simulink model "Microgrid_W"  (R2020a)
settings: Solver=ode15s  StartTime=0  StopTime=1440*1  MaxStep=1  RelTol=1e-3
libraries: simulink x4214, powerlib x685, simulink_extras x28, Microgrid_Library x18, powerlib_meascontrol x12
(part 2 of 48)

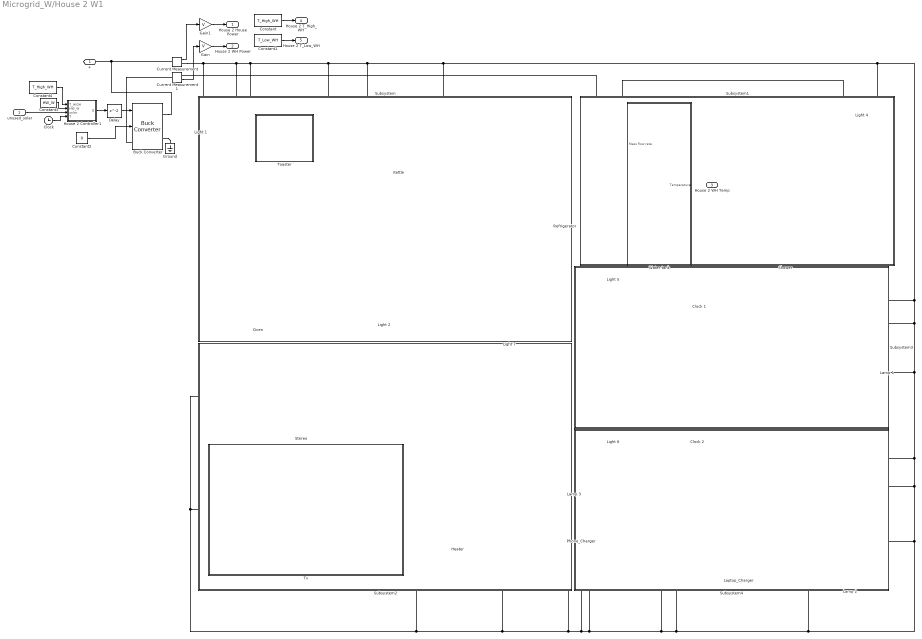
== system Microgrid_W/House 2 W1 ==
  unused_solar : Inport
  Buck Converter : powerlib/Power Electronics/Buck Converter  ModelType=Average model (D-controlled)  Ron=1e-3  Rs=1e6  Cs=inf  Vforward=[0,0]  Ron_Diode=1e-3  Rs_Diode=1e6  Cs_Diode=inf  Vf_Diode=1e-3  Rs_CurrentSource=inf
      settings: SourceProductBaseCode=PS
  Clock : Clock
  Clock 1 : Subsystem
      mask Display: image('Clock.jpg');
  Clock 2 : Subsystem
      mask Display: image('Clock.jpg');
  Constant : Constant  Value=T_High_WH
  Constant1 : Constant  Value=T_Low_WH
  Constant2 : Constant  Value=0
  Constant3 : Constant  Value=HW_W
  Constant4 : Constant  Value=T_High_WH
  Current Measurement : powerlib/Measurements/Current Measurement  PhasorSimulation=off  OutputType=Complex  PSBequivalent=0
  Current Measurement1 : powerlib/Measurements/Current Measurement  PhasorSimulation=off  OutputType=Complex  PSBequivalent=0
  Delay : Delay
  Gain : Gain  Gain=V
  Gain1 : Gain  Gain=V
  Ground : powerlib/Elements/Ground  LConnTagsString=a
  Heater : Subsystem
      mask Display: image('oil_heater.jpg');
  House 2 Controller1 : MATLAB Function  TreatAsAtomicUnit=on
  Kettle : Subsystem
      mask Display: image('jug.jpg');
  Lamp 1 : Subsystem
      mask Display: image('Lamp_1.jpg');
  Lamp 2 : Subsystem
      mask Display: image('Lamp_1.jpg');
  Lamp 3 : Subsystem
      mask Display: image('Lamp_1.jpg');
  Laptop_Charger : Subsystem
      mask Display: image('Laptop.jpg');
  Light 1 : Subsystem
      mask Display: image('LightBulb.jpg');
  Light 2 : Subsystem
      mask Display: image('Dishwasher.jpg');
  Light 4 : Subsystem
      mask Display: image('LightBulb.jpg');
  Light 5 : Subsystem
      mask Display: image('LightBulb.jpg');
  Light 6 : Subsystem
      mask Display: image('LightBulb.jpg');
  Light 7 : Subsystem
      mask Display: image('LightBulb.jpg');
  Oven : Subsystem
      mask Display: image('oven.jpg');
  Phone_Charger : Subsystem
      mask Display: image('Phone.jpg');
  Refrigerator : Subsystem
      mask Display: image('firdge1.JPG');
  Shower : Subsystem
      mask Display: image('Shower.jpg');
  Stereo : Subsystem
      mask Display: image('Stereo.jpg');
  Subsystem : Subsystem
      mask Display: patch([1 1 0 0],[1 0 0 1], [1, .4, .4])
  Subsystem1 : Subsystem
      mask Display: patch([1 1 0 0],[1 0 0 1], [0.6, .8, 1])
  Subsystem2 : Subsystem
      mask Display: patch([1 1 0 0],[1 0 0 1], [0.4, 1, .4])
  Subsystem3 : Subsystem
      mask Display: patch([1 1 0 0],[1 0 0 1], [0.8, 0.42, 0])
  Subsystem4 : Subsystem
      mask Display: patch([1 1 0 0],[1 0 0 1], [0.75, .75, .75])
  Toaster : Subsystem
      mask Display: image('toaster.jpg');
  Tv : Subsystem
      mask Display: image('Tel.jpg');
  Water tank : Subsystem
      mask Display: image('Hot Water.jpg');
  + : PMIOPort  Side=Left
  House 2 House Power : Outport
  House 2 WH Power : Outport  Port=2
  House 2 WH Temp : Outport  Port=3
  House 2 T_High_WH : Outport  Port=4
  House 2 T_Low_WH : Outport  Port=5
  wires:
  Shower/1(Out1) -> Water tank/1(Mass flow rate)
  Water tank/1(Temperature) -> House 2 WH Temp/1
  Constant/1 -> House 2 T_High_WH/1
  Constant1/1 -> House 2 T_Low_WH/1
  Current Measurement1/1 -> Gain/1
  Current Measurement/1 -> Gain1/1
  Gain1/1 -> House 2 House Power/1
  Constant2/1 -> Buck Converter/2
  Constant3/1 -> House 2 Controller1/2(HW_W)
  House 2 Controller1/1(D) -> Delay/1
  Delay/1 -> Buck Converter/1
  Clock/1 -> House 2 Controller1/4(T)
  unused_solar/1 -> House 2 Controller1/3(solar)
  Gain/1 -> House 2 WH Power/1
  Constant4/1 -> House 2 Controller1/1(T_HIGH)
  connections:
  Buck Converter/LConn1 -- Current Measurement1/LConn1
  Light 1/LConn1 -- Oven/LConn1 -- Current Measurement/RConn1 -- Light 4/LConn1 -- Light 5/LConn1 -- Clock 1/LConn1 -- Lamp 1/LConn1 -- Clock 2/LConn1 -- Light 6/LConn1 -- Lamp 2/LConn1 -- Laptop_Charger/RConn1 -- Laptop_Charger/LConn1 -- Phone_Charger/RConn1 -- Phone_Charger/LConn2 -- Phone_Charger/LConn1 -- Light 7/LConn1 -- Lamp 3/LConn1 -- Stereo/LConn1 -- Tv/LConn1 -- Heater/LConn1 -- Refrigerator/LConn1 -- Kettle/LConn1 -- Light 2/LConn1 -- Toaster/LConn1
  Water tank/LConn1 -- Current Measurement1/RConn1
  Current Measurement/LConn1 -- Buck Converter/RConn1 -- +/RConn1
  Buck Converter/RConn2 -- Ground/LConn1

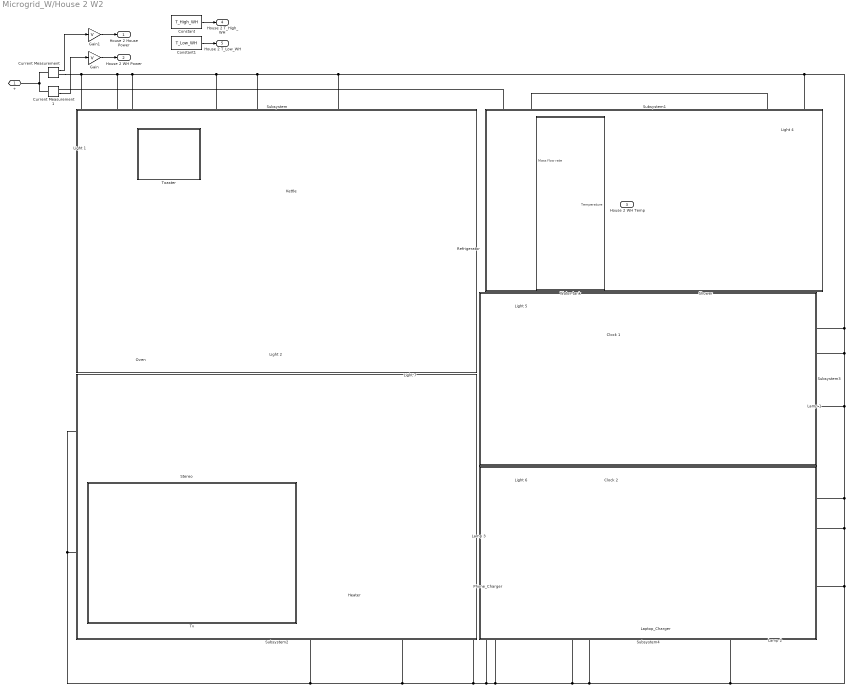
== system Microgrid_W/House 2 W2 ==
  Clock 1 : Subsystem
      mask Display: image('Clock.jpg');
  Clock 2 : Subsystem
      mask Display: image('Clock.jpg');
  Constant : Constant  Value=T_High_WH
  Constant1 : Constant  Value=T_Low_WH
  Current Measurement : powerlib/Measurements/Current Measurement  PhasorSimulation=off  OutputType=Complex  PSBequivalent=0
  Current Measurement1 : powerlib/Measurements/Current Measurement  PhasorSimulation=off  OutputType=Complex  PSBequivalent=0
  Gain : Gain  Gain=V
  Gain1 : Gain  Gain=V
  Heater : Subsystem
      mask Display: image('oil_heater.jpg');
  Kettle : Subsystem
      mask Display: image('jug.jpg');
  Lamp 1 : Subsystem
      mask Display: image('Lamp_1.jpg');
  Lamp 2 : Subsystem
      mask Display: image('Lamp_1.jpg');
  Lamp 3 : Subsystem
      mask Display: image('Lamp_1.jpg');
  Laptop_Charger : Subsystem
      mask Display: image('Laptop.jpg');
  Light 1 : Subsystem
      mask Display: image('LightBulb.jpg');
  Light 2 : Subsystem
      mask Display: image('Dishwasher.jpg');
  Light 4 : Subsystem
      mask Display: image('LightBulb.jpg');
  Light 5 : Subsystem
      mask Display: image('LightBulb.jpg');
  Light 6 : Subsystem
      mask Display: image('LightBulb.jpg');
  Light 7 : Subsystem
      mask Display: image('LightBulb.jpg');
  Oven : Subsystem
      mask Display: image('oven.jpg');
  Phone_Charger : Subsystem
      mask Display: image('Phone.jpg');
  Refrigerator : Subsystem
      mask Display: image('firdge1.JPG');
  Shower : Subsystem
      mask Display: image('Shower.jpg');
  Stereo : Subsystem
      mask Display: image('Stereo.jpg');
  Subsystem : Subsystem
      mask Display: patch([1 1 0 0],[1 0 0 1], [1, .4, .4])
  Subsystem1 : Subsystem
      mask Display: patch([1 1 0 0],[1 0 0 1], [0.6, .8, 1])
  Subsystem2 : Subsystem
      mask Display: patch([1 1 0 0],[1 0 0 1], [0.4, 1, .4])
  Subsystem3 : Subsystem
      mask Display: patch([1 1 0 0],[1 0 0 1], [0.8, 0.42, 0])
  Subsystem4 : Subsystem
      mask Display: patch([1 1 0 0],[1 0 0 1], [0.75, .75, .75])
  Toaster : Subsystem
      mask Display: image('toaster.jpg');
  Tv : Subsystem
      mask Display: image('Tel.jpg');
  Water tank : Subsystem
      mask Display: image('Hot Water.jpg');
  + : PMIOPort  Side=Left
  House 2 House Power : Outport
  House 2 WH Power : Outport  Port=2
  House 2 WH Temp : Outport  Port=3
  House 2 T_High_WH : Outport  Port=4
  House 2 T_Low_WH : Outport  Port=5
  wires:
  Shower/1(Out1) -> Water tank/1(Mass flow rate)
  Water tank/1(Temperature) -> House 2 WH Temp/1
  Constant/1 -> House 2 T_High_WH/1
  Constant1/1 -> House 2 T_Low_WH/1
  Current Measurement1/1 -> Gain/1
  Gain/1 -> House 2 WH Power/1
  Current Measurement/1 -> Gain1/1
  Gain1/1 -> House 2 House Power/1
  connections:
  Light 1/LConn1 -- Oven/LConn1 -- Current Measurement/RConn1 -- Light 4/LConn1 -- Light 5/LConn1 -- Clock 1/LConn1 -- Lamp 1/LConn1 -- Clock 2/LConn1 -- Light 6/LConn1 -- Lamp 2/LConn1 -- Laptop_Charger/RConn1 -- Laptop_Charger/LConn1 -- Phone_Charger/RConn1 -- Phone_Charger/LConn2 -- Phone_Charger/LConn1 -- Light 7/LConn1 -- Lamp 3/LConn1 -- Stereo/LConn1 -- Tv/LConn1 -- Heater/LConn1 -- Refrigerator/LConn1 -- Kettle/LConn1 -- Light 2/LConn1 -- Toaster/LConn1
  Water tank/LConn1 -- Current Measurement1/RConn1
  Current Measurement1/LConn1 -- Current Measurement/LConn1 -- +/RConn1

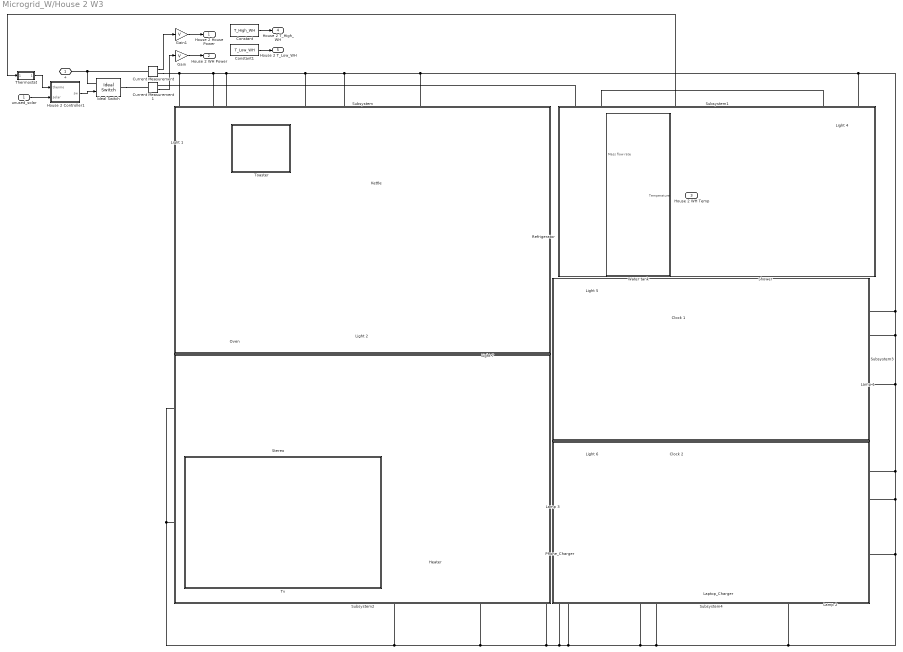
== system Microgrid_W/House 2 W3 ==
  unused_solar : Inport
  Clock 1 : Subsystem
      mask Display: image('Clock.jpg');
  Clock 2 : Subsystem
      mask Display: image('Clock.jpg');
  Constant : Constant  Value=T_High_WH
  Constant1 : Constant  Value=T_Low_WH
  Current Measurement : powerlib/Measurements/Current Measurement  PhasorSimulation=off  OutputType=Complex  PSBequivalent=0
  Current Measurement1 : powerlib/Measurements/Current Measurement  PhasorSimulation=off  OutputType=Complex  PSBequivalent=0
  Gain : Gain  Gain=V
  Gain1 : Gain  Gain=V
  Heater : Subsystem
      mask Display: image('oil_heater.jpg');
  House 2 Controller1 : MATLAB Function  TreatAsAtomicUnit=on
  Ideal Switch : powerlib/Power Electronics/Ideal Switch  Ron=0  Lon=0  IC=0  Rs=1e5  Cs=inf  Measurements=off
  Kettle : Subsystem
      mask Display: image('jug.jpg');
  Lamp 1 : Subsystem
      mask Display: image('Lamp_1.jpg');
  Lamp 2 : Subsystem
      mask Display: image('Lamp_1.jpg');
  Lamp 3 : Subsystem
      mask Display: image('Lamp_1.jpg');
  Laptop_Charger : Subsystem
      mask Display: image('Laptop.jpg');
  Light 1 : Subsystem
      mask Display: image('LightBulb.jpg');
  Light 2 : Subsystem
      mask Display: image('Dishwasher.jpg');
  Light 4 : Subsystem
      mask Display: image('LightBulb.jpg');
  Light 5 : Subsystem
      mask Display: image('LightBulb.jpg');
  Light 6 : Subsystem
      mask Display: image('LightBulb.jpg');
  Light 7 : Subsystem
      mask Display: image('LightBulb.jpg');
  Oven : Subsystem
      mask Display: image('oven.jpg');
  Phone_Charger : Subsystem
      mask Display: image('Phone.jpg');
  Refrigerator : Subsystem
      mask Display: image('firdge1.JPG');
  Shower : Subsystem
      mask Display: image('Shower.jpg');
  Stereo : Subsystem
      mask Display: image('Stereo.jpg');
  Subsystem : Subsystem
      mask Display: patch([1 1 0 0],[1 0 0 1], [1, .4, .4])
  Subsystem1 : Subsystem
      mask Display: patch([1 1 0 0],[1 0 0 1], [0.6, .8, 1])
  Subsystem2 : Subsystem
      mask Display: patch([1 1 0 0],[1 0 0 1], [0.4, 1, .4])
  Subsystem3 : Subsystem
      mask Display: patch([1 1 0 0],[1 0 0 1], [0.8, 0.42, 0])
  Subsystem4 : Subsystem
      mask Display: patch([1 1 0 0],[1 0 0 1], [0.75, .75, .75])
  Thermostat : Subsystem
  Toaster : Subsystem
      mask Display: image('toaster.jpg');
  Tv : Subsystem
      mask Display: image('Tel.jpg');
  Water tank : Subsystem
      mask Display: image('Hot Water.jpg');
  + : PMIOPort  Side=Left
  House 2 House Power : Outport
  House 2 WH Power : Outport  Port=2
  House 2 WH Temp : Outport  Port=3
  House 2 T_High_WH : Outport  Port=4
  House 2 T_Low_WH : Outport  Port=5
  wires:
  Gain1/1 -> House 2 House Power/1
  Current Measurement/1 -> Gain1/1
  Gain/1 -> House 2 WH Power/1
  Current Measurement1/1 -> Gain/1
  Constant1/1 -> House 2 T_Low_WH/1
  Constant/1 -> House 2 T_High_WH/1
  Water tank/1(Temperature) -> Thermostat/1(In1), House 2 WH Temp/1
  Shower/1(Out1) -> Water tank/1(Mass flow rate)
  House 2 Controller1/1(sw) -> Ideal Switch/1
  unused_solar/1 -> House 2 Controller1/2(solar)
  Thermostat/1(Out1) -> House 2 Controller1/1(thermo)
  connections:
  +/RConn1 -- Current Measurement/LConn1 -- Ideal Switch/LConn1
  Water tank/LConn1 -- Current Measurement1/RConn1
  Toaster/LConn1 -- Light 2/LConn1 -- Kettle/LConn1 -- Refrigerator/LConn1 -- Heater/LConn1 -- Tv/LConn1 -- Stereo/LConn1 -- Lamp 3/LConn1 -- Light 7/LConn1 -- Phone_Charger/LConn1 -- Phone_Charger/LConn2 -- Phone_Charger/RConn1 -- Laptop_Charger/LConn1 -- Laptop_Charger/RConn1 -- Lamp 2/LConn1 -- Light 6/LConn1 -- Clock 2/LConn1 -- Lamp 1/LConn1 -- Clock 1/LConn1 -- Light 5/LConn1 -- Light 4/LConn1 -- Current Measurement/RConn1 -- Oven/LConn1 -- Light 1/LConn1
  Ideal Switch/RConn1 -- Current Measurement1/LConn1

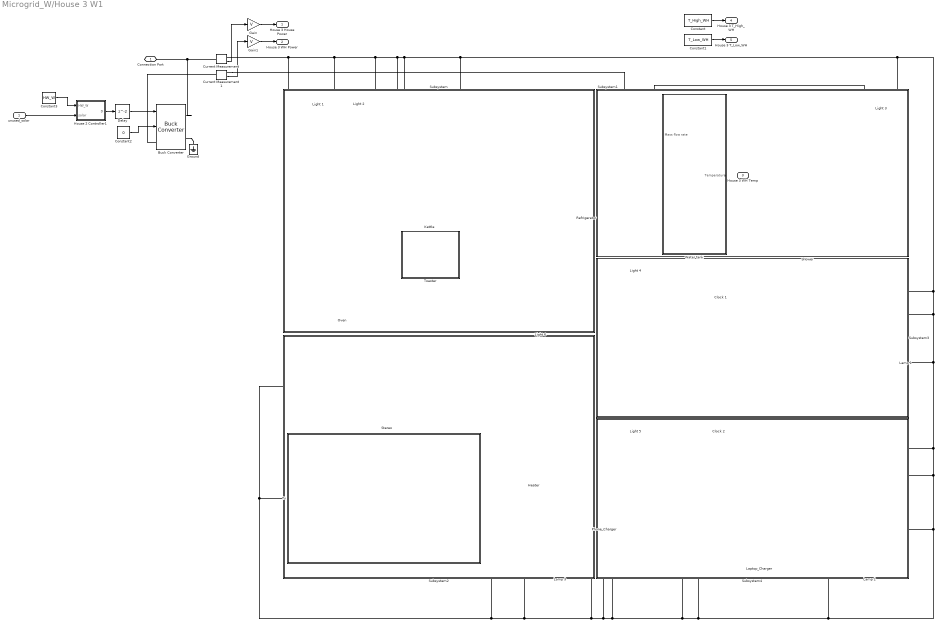
== system Microgrid_W/House 3 W1 ==
  unused_solar : Inport
  Buck Converter : powerlib/Power Electronics/Buck Converter  ModelType=Average model (D-controlled)  Ron=1e-3  Rs=1e6  Cs=inf  Vforward=[0,0]  Ron_Diode=1e-3  Rs_Diode=1e6  Cs_Diode=inf  Vf_Diode=1e-3  Rs_CurrentSource=inf
      settings: SourceProductBaseCode=PS
  Clock 1 : Subsystem
      mask Display: image('Clock.jpg');
  Clock 2 : Subsystem
      mask Display: image('Clock.jpg');
  Constant : Constant  Value=T_High_WH
  Constant1 : Constant  Value=T_Low_WH
  Constant2 : Constant  Value=0
  Constant3 : Constant  Value=HW_W
  Current Measurement : powerlib/Measurements/Current Measurement  PhasorSimulation=off  OutputType=Complex  PSBequivalent=0
  Current Measurement1 : powerlib/Measurements/Current Measurement  PhasorSimulation=off  OutputType=Complex  PSBequivalent=0
  Delay : Delay
  Gain : Gain  Gain=V
  Gain1 : Gain  Gain=V
  Ground : powerlib/Elements/Ground  LConnTagsString=a
  Heater : Subsystem
      mask Display: image('oil_heater.jpg');
  House 2 Controller1 : MATLAB Function  TreatAsAtomicUnit=on
  Kettle : Subsystem
      mask Display: image('jug.jpg');
  Lamp 1 : Subsystem
      mask Display: image('Lamp_1.jpg');
  Lamp 2 : Subsystem
      mask Display: image('Lamp_1.jpg');
  Lamp 3 : Subsystem
      mask Display: image('Lamp_1.jpg');
  Laptop_Charger : Subsystem
      mask Display: image('Laptop.jpg');
  Light 1 : Subsystem
      mask Display: image('LightBulb.jpg');
  Light 2 : Subsystem
      mask Display: image('LightBulb.jpg');
  Light 3 : Subsystem
      mask Display: image('LightBulb.jpg');
  Light 4 : Subsystem
      mask Display: image('LightBulb.jpg');
  Light 5 : Subsystem
      mask Display: image('LightBulb.jpg');
  Light 6 : Subsystem
      mask Display: image('LightBulb.jpg');
  Oven : Subsystem
      mask Display: image('oven.jpg');
  Phone_Charger : Subsystem
      mask Display: image('Phone.jpg');
  Refrigerator : Subsystem
      mask Display: image('firdge1.JPG');
  Shower : Subsystem
      mask Display: image('Shower.jpg');
  Stereo : Subsystem
      mask Display: image('Stereo.jpg');
  Subsystem : Subsystem
      mask Display: patch([1 1 0 0],[1 0 0 1], [1, .4, .4])
  Subsystem1 : Subsystem
      mask Display: patch([1 1 0 0],[1 0 0 1], [0.6, .8, 1])
  Subsystem2 : Subsystem
      mask Display: patch([1 1 0 0],[1 0 0 1], [0.4, 1, .4])
  Subsystem3 : Subsystem
      mask Display: patch([1 1 0 0],[1 0 0 1], [0.8, 0.42, 0])
  Subsystem4 : Subsystem
      mask Display: patch([1 1 0 0],[1 0 0 1], [0.75, .75, .75])
  Toaster : Subsystem
      mask Display: image('toaster.jpg');
  Tv : Subsystem
      mask Display: image('Tel.jpg');
  Water tank : Subsystem
      mask Display: image('Hot Water.jpg');
  Connection Port : PMIOPort  Side=Left
  House 3 House Power : Outport
  House 3 WH Power : Outport  Port=2
  House 3 WH Temp : Outport  Port=3
  House 3 T_High_WH : Outport  Port=4
  House 3 T_Low_WH : Outport  Port=5
  wires:
  Water tank/1(Temperature) -> House 3 WH Temp/1
  Shower/1(Out1) -> Water tank/1(Mass flow rate)
  Constant/1 -> House 3 T_High_WH/1
  Constant1/1 -> House 3 T_Low_WH/1
  Current Measurement/1 -> Gain/1
  Current Measurement1/1 -> Gain1/1
  Gain1/1 -> House 3 WH Power/1
  Gain/1 -> House 3 House Power/1
  Constant2/1 -> Buck Converter/2
  unused_solar/1 -> House 2 Controller1/2(solar)
  House 2 Controller1/1(D) -> Delay/1
  Constant3/1 -> House 2 Controller1/1(HW_W)
  Delay/1 -> Buck Converter/1
  connections:
  Light 3/LConn1 -- Light 4/LConn1 -- Clock 1/LConn1 -- Lamp 1/LConn1 -- Clock 2/LConn1 -- Light 5/LConn1 -- Lamp 2/LConn1 -- Laptop_Charger/RConn1 -- Laptop_Charger/LConn1 -- Phone_Charger/RConn1 -- Phone_Charger/LConn2 -- Phone_Charger/LConn1 -- Light 6/LConn1 -- Lamp 3/LConn1 -- Heater/LConn1 -- Stereo/LConn1 -- Tv/LConn1 -- Current Measurement/RConn1 -- Oven/LConn1 -- Light 1/LConn1 -- Light 2/LConn1 -- Toaster/LConn1 -- Kettle/LConn1 -- Refrigerator/LConn1
  Current Measurement/LConn1 -- Buck Converter/RConn1 -- Connection Port/RConn1
  Current Measurement1/RConn1 -- Water tank/LConn1
  Buck Converter/RConn2 -- Ground/LConn1
  Buck Converter/LConn1 -- Current Measurement1/LConn1

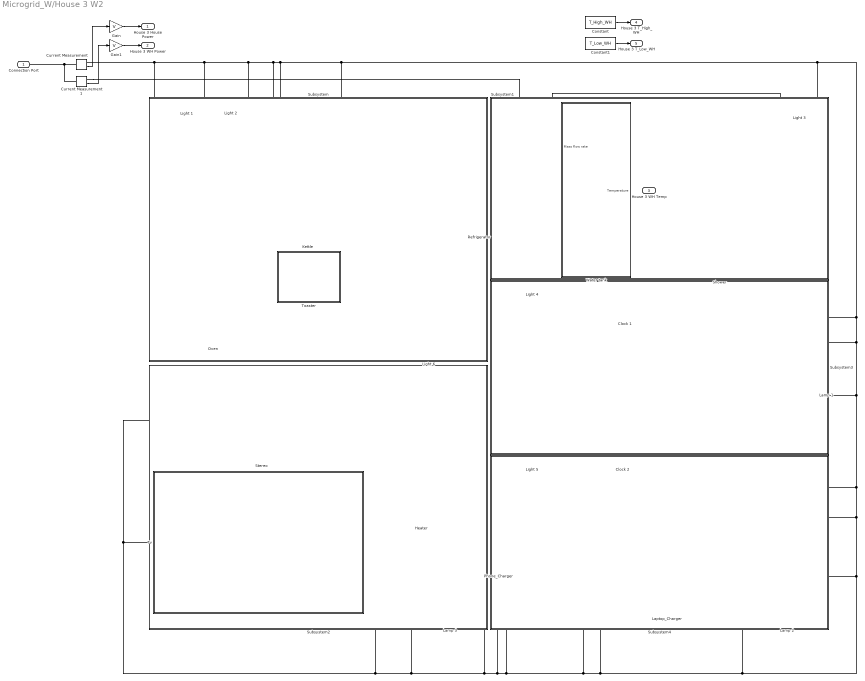
== system Microgrid_W/House 3 W2 ==
  Clock 1 : Subsystem
      mask Display: image('Clock.jpg');
  Clock 2 : Subsystem
      mask Display: image('Clock.jpg');
  Constant : Constant  Value=T_High_WH
  Constant1 : Constant  Value=T_Low_WH
  Current Measurement : powerlib/Measurements/Current Measurement  PhasorSimulation=off  OutputType=Complex  PSBequivalent=0
  Current Measurement1 : powerlib/Measurements/Current Measurement  PhasorSimulation=off  OutputType=Complex  PSBequivalent=0
  Gain : Gain  Gain=V
  Gain1 : Gain  Gain=V
  Heater : Subsystem
      mask Display: image('oil_heater.jpg');
  Kettle : Subsystem
      mask Display: image('jug.jpg');
  Lamp 1 : Subsystem
      mask Display: image('Lamp_1.jpg');
  Lamp 2 : Subsystem
      mask Display: image('Lamp_1.jpg');
  Lamp 3 : Subsystem
      mask Display: image('Lamp_1.jpg');
  Laptop_Charger : Subsystem
      mask Display: image('Laptop.jpg');
  Light 1 : Subsystem
      mask Display: image('LightBulb.jpg');
  Light 2 : Subsystem
      mask Display: image('LightBulb.jpg');
  Light 3 : Subsystem
      mask Display: image('LightBulb.jpg');
  Light 4 : Subsystem
      mask Display: image('LightBulb.jpg');
  Light 5 : Subsystem
      mask Display: image('LightBulb.jpg');
  Light 6 : Subsystem
      mask Display: image('LightBulb.jpg');
  Oven : Subsystem
      mask Display: image('oven.jpg');
  Phone_Charger : Subsystem
      mask Display: image('Phone.jpg');
  Refrigerator : Subsystem
      mask Display: image('firdge1.JPG');
  Shower : Subsystem
      mask Display: image('Shower.jpg');
  Stereo : Subsystem
      mask Display: image('Stereo.jpg');
  Subsystem : Subsystem
      mask Display: patch([1 1 0 0],[1 0 0 1], [1, .4, .4])
  Subsystem1 : Subsystem
      mask Display: patch([1 1 0 0],[1 0 0 1], [0.6, .8, 1])
  Subsystem2 : Subsystem
      mask Display: patch([1 1 0 0],[1 0 0 1], [0.4, 1, .4])
  Subsystem3 : Subsystem
      mask Display: patch([1 1 0 0],[1 0 0 1], [0.8, 0.42, 0])
  Subsystem4 : Subsystem
      mask Display: patch([1 1 0 0],[1 0 0 1], [0.75, .75, .75])
  Toaster : Subsystem
      mask Display: image('toaster.jpg');
  Tv : Subsystem
      mask Display: image('Tel.jpg');
  Water tank : Subsystem
      mask Display: image('Hot Water.jpg');
  Connection Port : PMIOPort  Side=Left
  House 3 House Power : Outport
  House 3 WH Power : Outport  Port=2
  House 3 WH Temp : Outport  Port=3
  House 3 T_High_WH : Outport  Port=4
  House 3 T_Low_WH : Outport  Port=5
  wires:
  Shower/1(Out1) -> Water tank/1(Mass flow rate)
  Water tank/1(Temperature) -> House 3 WH Temp/1
  Constant/1 -> House 3 T_High_WH/1
  Constant1/1 -> House 3 T_Low_WH/1
  Current Measurement/1 -> Gain/1
  Current Measurement1/1 -> Gain1/1
  Gain1/1 -> House 3 WH Power/1
  Gain/1 -> House 3 House Power/1
  connections:
  Light 3/LConn1 -- Light 4/LConn1 -- Clock 1/LConn1 -- Lamp 1/LConn1 -- Clock 2/LConn1 -- Light 5/LConn1 -- Lamp 2/LConn1 -- Laptop_Charger/RConn1 -- Laptop_Charger/LConn1 -- Phone_Charger/RConn1 -- Phone_Charger/LConn2 -- Phone_Charger/LConn1 -- Light 6/LConn1 -- Lamp 3/LConn1 -- Heater/LConn1 -- Stereo/LConn1 -- Tv/LConn1 -- Current Measurement/RConn1 -- Oven/LConn1 -- Light 1/LConn1 -- Light 2/LConn1 -- Toaster/LConn1 -- Kettle/LConn1 -- Refrigerator/LConn1
  Current Measurement/LConn1 -- Current Measurement1/LConn1 -- Connection Port/RConn1
  Current Measurement1/RConn1 -- Water tank/LConn1

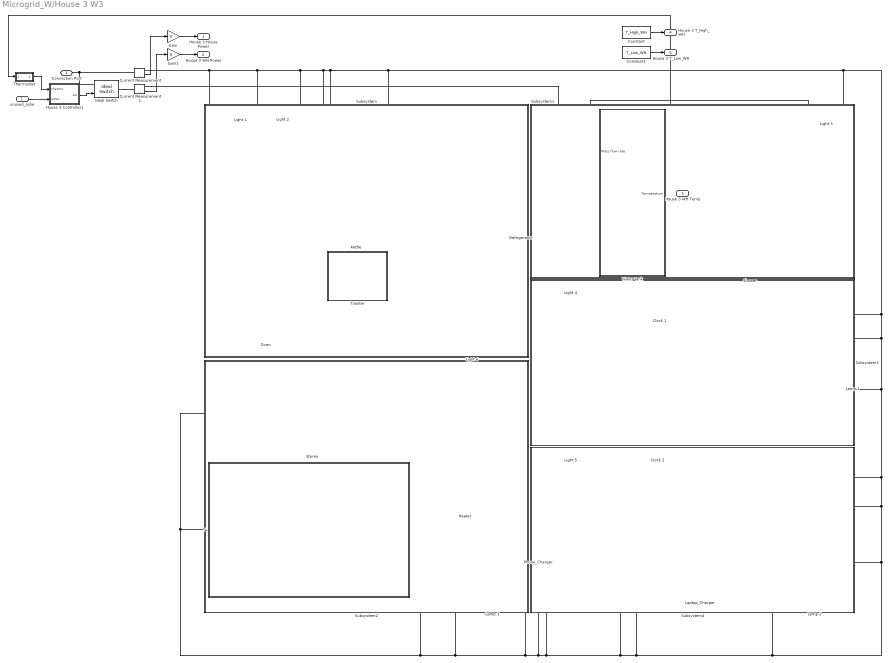
== system Microgrid_W/House 3 W3 ==
  unused_solar : Inport
  Clock 1 : Subsystem
      mask Display: image('Clock.jpg');
  Clock 2 : Subsystem
      mask Display: image('Clock.jpg');
  Constant : Constant  Value=T_High_WH
  Constant1 : Constant  Value=T_Low_WH
  Current Measurement : powerlib/Measurements/Current Measurement  PhasorSimulation=off  OutputType=Complex  PSBequivalent=0
  Current Measurement1 : powerlib/Measurements/Current Measurement  PhasorSimulation=off  OutputType=Complex  PSBequivalent=0
  Gain : Gain  Gain=V
  Gain1 : Gain  Gain=V
  Heater : Subsystem
      mask Display: image('oil_heater.jpg');
  House 3 Controller1 : MATLAB Function  TreatAsAtomicUnit=on
  Ideal Switch : powerlib/Power Electronics/Ideal Switch  Ron=0  Lon=0  IC=0  Rs=1e5  Cs=inf  Measurements=off
  Kettle : Subsystem
      mask Display: image('jug.jpg');
  Lamp 1 : Subsystem
      mask Display: image('Lamp_1.jpg');
  Lamp 2 : Subsystem
      mask Display: image('Lamp_1.jpg');
  Lamp 3 : Subsystem
      mask Display: image('Lamp_1.jpg');
  Laptop_Charger : Subsystem
      mask Display: image('Laptop.jpg');
  Light 1 : Subsystem
      mask Display: image('LightBulb.jpg');
  Light 2 : Subsystem
      mask Display: image('LightBulb.jpg');
  Light 3 : Subsystem
      mask Display: image('LightBulb.jpg');
  Light 4 : Subsystem
      mask Display: image('LightBulb.jpg');
  Light 5 : Subsystem
      mask Display: image('LightBulb.jpg');
  Light 6 : Subsystem
      mask Display: image('LightBulb.jpg');
  Oven : Subsystem
      mask Display: image('oven.jpg');
  Phone_Charger : Subsystem
      mask Display: image('Phone.jpg');
  Refrigerator : Subsystem
      mask Display: image('firdge1.JPG');
  Shower : Subsystem
      mask Display: image('Shower.jpg');
  Stereo : Subsystem
      mask Display: image('Stereo.jpg');
  Subsystem : Subsystem
      mask Display: patch([1 1 0 0],[1 0 0 1], [1, .4, .4])
  Subsystem1 : Subsystem
      mask Display: patch([1 1 0 0],[1 0 0 1], [0.6, .8, 1])
  Subsystem2 : Subsystem
      mask Display: patch([1 1 0 0],[1 0 0 1], [0.4, 1, .4])
  Subsystem3 : Subsystem
      mask Display: patch([1 1 0 0],[1 0 0 1], [0.8, 0.42, 0])
  Subsystem4 : Subsystem
      mask Display: patch([1 1 0 0],[1 0 0 1], [0.75, .75, .75])
  Thermostat : Subsystem
  Toaster : Subsystem
      mask Display: image('toaster.jpg');
  Tv : Subsystem
      mask Display: image('Tel.jpg');
  Water tank : Subsystem
      mask Display: image('Hot Water.jpg');
  Connection Port : PMIOPort  Side=Left
  House 3 House Power : Outport
  House 3 WH Power : Outport  Port=2
  House 3 WH Temp : Outport  Port=3
  House 3 T_High_WH : Outport  Port=4
  House 3 T_Low_WH : Outport  Port=5
  wires:
  Gain/1 -> House 3 House Power/1
  Gain1/1 -> House 3 WH Power/1
  Current Measurement1/1 -> Gain1/1
  Current Measurement/1 -> Gain/1
  Constant1/1 -> House 3 T_Low_WH/1
  Constant/1 -> House 3 T_High_WH/1
  Shower/1(Out1) -> Water tank/1(Mass flow rate)
  Water tank/1(Temperature) -> Thermostat/1(In1), House 3 WH Temp/1
  unused_solar/1 -> House 3 Controller1/2(solar)
  Thermostat/1(Out1) -> House 3 Controller1/1(thermo)
  House 3 Controller1/1(sw) -> Ideal Switch/1
  connections:
  Current Measurement1/RConn1 -- Water tank/LConn1
  Current Measurement/LConn1 -- Ideal Switch/LConn1 -- Connection Port/RConn1
  Refrigerator/LConn1 -- Kettle/LConn1 -- Toaster/LConn1 -- Light 2/LConn1 -- Light 1/LConn1 -- Oven/LConn1 -- Current Measurement/RConn1 -- Tv/LConn1 -- Stereo/LConn1 -- Heater/LConn1 -- Lamp 3/LConn1 -- Light 6/LConn1 -- Phone_Charger/LConn1 -- Phone_Charger/LConn2 -- Phone_Charger/RConn1 -- Laptop_Charger/LConn1 -- Laptop_Charger/RConn1 -- Lamp 2/LConn1 -- Light 5/LConn1 -- Clock 2/LConn1 -- Lamp 1/LConn1 -- Clock 1/LConn1 -- Light 4/LConn1 -- Light 3/LConn1
  Ideal Switch/RConn1 -- Current Measurement1/LConn1

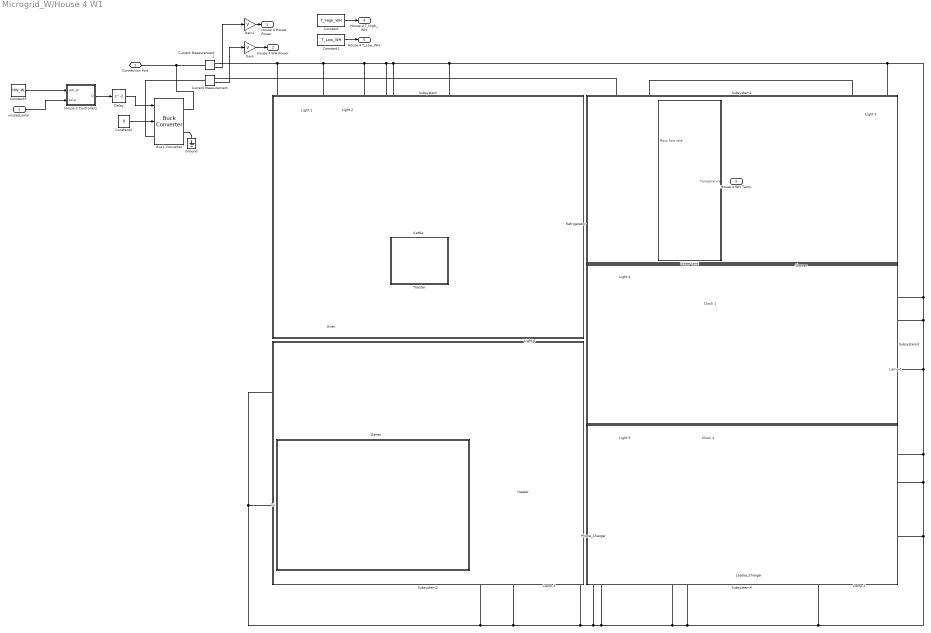
== system Microgrid_W/House 4 W1 ==
  unused_solar : Inport
  Buck Converter : powerlib/Power Electronics/Buck Converter  ModelType=Average model (D-controlled)  Ron=1e-3  Rs=1e6  Cs=inf  Vforward=[0,0]  Ron_Diode=1e-3  Rs_Diode=1e6  Cs_Diode=inf  Vf_Diode=1e-3  Rs_CurrentSource=inf
      settings: SourceProductBaseCode=PS
  Clock 1 : Subsystem
      mask Display: image('Clock.jpg');
  Clock 2 : Subsystem
      mask Display: image('Clock.jpg');
  Constant : Constant  Value=T_High_WH
  Constant1 : Constant  Value=T_Low_WH
  Constant2 : Constant  Value=0
  Constant3 : Constant  Value=HW_W
  Current Measurement : powerlib/Measurements/Current Measurement  PhasorSimulation=off  OutputType=Complex  PSBequivalent=0
  Current Measurement1 : powerlib/Measurements/Current Measurement  PhasorSimulation=off  OutputType=Complex  PSBequivalent=0
  Delay : Delay
  Gain : Gain  Gain=V
  Gain1 : Gain  Gain=V
  Ground : powerlib/Elements/Ground  LConnTagsString=a
  Heater : Subsystem
      mask Display: image('oil_heater.jpg');
  House 2 Controller1 : MATLAB Function  TreatAsAtomicUnit=on
  Kettle : Subsystem
      mask Display: image('jug.jpg');
  Lamp 1 : Subsystem
      mask Display: image('Lamp_1.jpg');
  Lamp 2 : Subsystem
      mask Display: image('Lamp_1.jpg');
  Lamp 3 : Subsystem
      mask Display: image('Lamp_1.jpg');
  Laptop_Charger : Subsystem
      mask Display: image('Laptop.jpg');
  Light 1 : Subsystem
      mask Display: image('LightBulb.jpg');
  Light 2 : Subsystem
      mask Display: image('LightBulb.jpg');
  Light 3 : Subsystem
      mask Display: image('LightBulb.jpg');
  Light 4 : Subsystem
      mask Display: image('LightBulb.jpg');
  Light 5 : Subsystem
      mask Display: image('LightBulb.jpg');
  Light 6 : Subsystem
      mask Display: image('LightBulb.jpg');
  Oven : Subsystem
      mask Display: image('oven.jpg');
  Phone_Charger : Subsystem
      mask Display: image('Phone.jpg');
  Refrigerator : Subsystem
      mask Display: image('firdge1.JPG');
  Shower : Subsystem
      mask Display: image('Shower.jpg');
  Stereo : Subsystem
      mask Display: image('Stereo.jpg');
  Subsystem : Subsystem
      mask Display: patch([1 1 0 0],[1 0 0 1], [1, .4, .4])
  Subsystem1 : Subsystem
      mask Display: patch([1 1 0 0],[1 0 0 1], [0.6, .8, 1])
  Subsystem2 : Subsystem
      mask Display: patch([1 1 0 0],[1 0 0 1], [0.4, 1, .4])
  Subsystem3 : Subsystem
      mask Display: patch([1 1 0 0],[1 0 0 1], [0.8, 0.42, 0])
  Subsystem4 : Subsystem
      mask Display: patch([1 1 0 0],[1 0 0 1], [0.75, .75, .75])
  Toaster : Subsystem
      mask Display: image('toaster.jpg');
  Tv : Subsystem
      mask Display: image('Tel.jpg');
  Water tank : Subsystem
      mask Display: image('Hot Water.jpg');
  Connection Port : PMIOPort  Side=Left
  House 4 House Power : Outport
  House 4 WH Power : Outport  Port=2
  House 4 WH Temp : Outport  Port=3
  House 4 T_High_WH : Outport  Port=4
  House 4 T_Low_WH : Outport  Port=5
  wires:
  Shower/1(Out1) -> Water tank/1(Mass flow rate)
  Water tank/1(Temperature) -> House 4 WH Temp/1
  Current Measurement/1 -> Gain/1
  Constant/1 -> House 4 T_High_WH/1
  Constant1/1 -> House 4 T_Low_WH/1
  Gain/1 -> House 4 WH Power/1
  Gain1/1 -> House 4 House Power/1
  Current Measurement1/1 -> Gain1/1
  Constant3/1 -> House 2 Controller1/1(HW_W)
  Constant2/1 -> Buck Converter/2
  unused_solar/1 -> House 2 Controller1/2(solar)
  House 2 Controller1/1(D) -> Delay/1
  Delay/1 -> Buck Converter/1
  connections:
  Tv/LConn1 -- Stereo/LConn1 -- Heater/LConn1 -- Lamp 3/LConn1 -- Light 6/LConn1 -- Phone_Charger/LConn1 -- Phone_Charger/LConn2 -- Phone_Charger/RConn1 -- Laptop_Charger/LConn1 -- Laptop_Charger/RConn1 -- Lamp 2/LConn1 -- Light 5/LConn1 -- Clock 2/LConn1 -- Lamp 1/LConn1 -- Clock 1/LConn1 -- Light 4/LConn1 -- Light 3/LConn1 -- Current Measurement1/RConn1 -- Oven/LConn1 -- Light 1/LConn1 -- Light 2/LConn1 -- Toaster/LConn1 -- Kettle/LConn1 -- Refrigerator/LConn1
  Water tank/LConn1 -- Current Measurement/RConn1
  Current Measurement1/LConn1 -- Buck Converter/RConn1 -- Connection Port/RConn1
  Buck Converter/LConn1 -- Current Measurement/LConn1
  Buck Converter/RConn2 -- Ground/LConn1

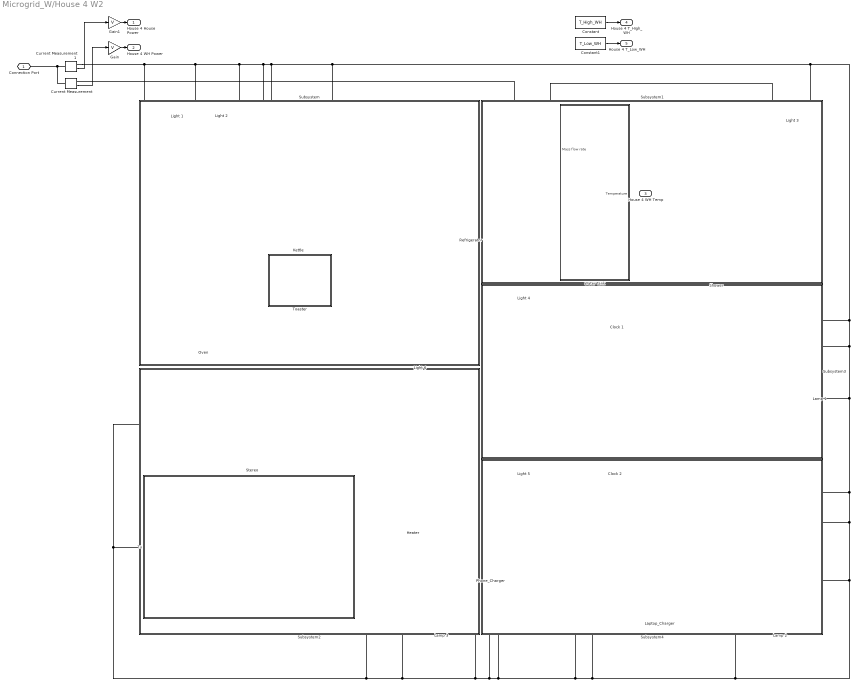
== system Microgrid_W/House 4 W2 ==
  Clock 1 : Subsystem
      mask Display: image('Clock.jpg');
  Clock 2 : Subsystem
      mask Display: image('Clock.jpg');
  Constant : Constant  Value=T_High_WH
  Constant1 : Constant  Value=T_Low_WH
  Current Measurement : powerlib/Measurements/Current Measurement  PhasorSimulation=off  OutputType=Complex  PSBequivalent=0
  Current Measurement1 : powerlib/Measurements/Current Measurement  PhasorSimulation=off  OutputType=Complex  PSBequivalent=0
  Gain : Gain  Gain=V
  Gain1 : Gain  Gain=V
  Heater : Subsystem
      mask Display: image('oil_heater.jpg');
  Kettle : Subsystem
      mask Display: image('jug.jpg');
  Lamp 1 : Subsystem
      mask Display: image('Lamp_1.jpg');
  Lamp 2 : Subsystem
      mask Display: image('Lamp_1.jpg');
  Lamp 3 : Subsystem
      mask Display: image('Lamp_1.jpg');
  Laptop_Charger : Subsystem
      mask Display: image('Laptop.jpg');
  Light 1 : Subsystem
      mask Display: image('LightBulb.jpg');
  Light 2 : Subsystem
      mask Display: image('LightBulb.jpg');
  Light 3 : Subsystem
      mask Display: image('LightBulb.jpg');
  Light 4 : Subsystem
      mask Display: image('LightBulb.jpg');
  Light 5 : Subsystem
      mask Display: image('LightBulb.jpg');
  Light 6 : Subsystem
      mask Display: image('LightBulb.jpg');
  Oven : Subsystem
      mask Display: image('oven.jpg');
  Phone_Charger : Subsystem
      mask Display: image('Phone.jpg');
  Refrigerator : Subsystem
      mask Display: image('firdge1.JPG');
  Shower : Subsystem
      mask Display: image('Shower.jpg');
  Stereo : Subsystem
      mask Display: image('Stereo.jpg');
  Subsystem : Subsystem
      mask Display: patch([1 1 0 0],[1 0 0 1], [1, .4, .4])
  Subsystem1 : Subsystem
      mask Display: patch([1 1 0 0],[1 0 0 1], [0.6, .8, 1])
  Subsystem2 : Subsystem
      mask Display: patch([1 1 0 0],[1 0 0 1], [0.4, 1, .4])
  Subsystem3 : Subsystem
      mask Display: patch([1 1 0 0],[1 0 0 1], [0.8, 0.42, 0])
  Subsystem4 : Subsystem
      mask Display: patch([1 1 0 0],[1 0 0 1], [0.75, .75, .75])
  Toaster : Subsystem
      mask Display: image('toaster.jpg');
  Tv : Subsystem
      mask Display: image('Tel.jpg');
  Water tank : Subsystem
      mask Display: image('Hot Water.jpg');
  Connection Port : PMIOPort  Side=Left
  House 4 House Power : Outport
  House 4 WH Power : Outport  Port=2
  House 4 WH Temp : Outport  Port=3
  House 4 T_High_WH : Outport  Port=4
  House 4 T_Low_WH : Outport  Port=5
  wires:
  Shower/1(Out1) -> Water tank/1(Mass flow rate)
  Water tank/1(Temperature) -> House 4 WH Temp/1
  Current Measurement/1 -> Gain/1
  Constant/1 -> House 4 T_High_WH/1
  Constant1/1 -> House 4 T_Low_WH/1
  Gain/1 -> House 4 WH Power/1
  Gain1/1 -> House 4 House Power/1
  Current Measurement1/1 -> Gain1/1
  connections:
  Tv/LConn1 -- Stereo/LConn1 -- Heater/LConn1 -- Lamp 3/LConn1 -- Light 6/LConn1 -- Phone_Charger/LConn1 -- Phone_Charger/LConn2 -- Phone_Charger/RConn1 -- Laptop_Charger/LConn1 -- Laptop_Charger/RConn1 -- Lamp 2/LConn1 -- Light 5/LConn1 -- Clock 2/LConn1 -- Lamp 1/LConn1 -- Clock 1/LConn1 -- Light 4/LConn1 -- Light 3/LConn1 -- Current Measurement1/RConn1 -- Oven/LConn1 -- Light 1/LConn1 -- Light 2/LConn1 -- Toaster/LConn1 -- Kettle/LConn1 -- Refrigerator/LConn1
  Water tank/LConn1 -- Current Measurement/RConn1
  Current Measurement/LConn1 -- Connection Port/RConn1 -- Current Measurement1/LConn1

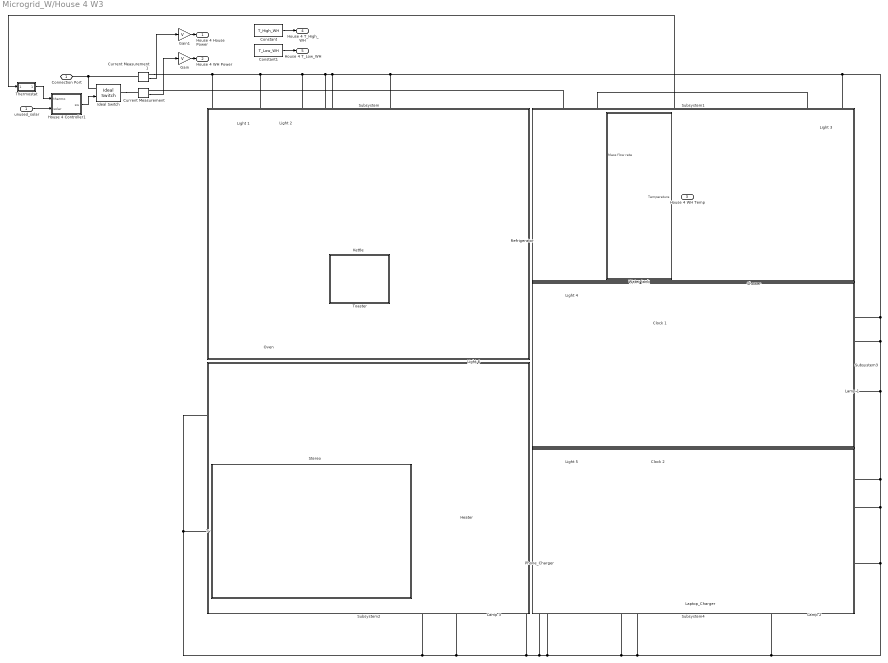
== system Microgrid_W/House 4 W3 ==
  unused_solar : Inport
  Clock 1 : Subsystem
      mask Display: image('Clock.jpg');
  Clock 2 : Subsystem
      mask Display: image('Clock.jpg');
  Constant : Constant  Value=T_High_WH
  Constant1 : Constant  Value=T_Low_WH
  Current Measurement : powerlib/Measurements/Current Measurement  PhasorSimulation=off  OutputType=Complex  PSBequivalent=0
  Current Measurement1 : powerlib/Measurements/Current Measurement  PhasorSimulation=off  OutputType=Complex  PSBequivalent=0
  Gain : Gain  Gain=V
  Gain1 : Gain  Gain=V
  Heater : Subsystem
      mask Display: image('oil_heater.jpg');
  House 4 Controller1 : MATLAB Function  TreatAsAtomicUnit=on
  Ideal Switch : powerlib/Power Electronics/Ideal Switch  Ron=0  Lon=0  IC=0  Rs=1e5  Cs=inf  Measurements=off
  Kettle : Subsystem
      mask Display: image('jug.jpg');
  Lamp 1 : Subsystem
      mask Display: image('Lamp_1.jpg');
  Lamp 2 : Subsystem
      mask Display: image('Lamp_1.jpg');
  Lamp 3 : Subsystem
      mask Display: image('Lamp_1.jpg');
  Laptop_Charger : Subsystem
      mask Display: image('Laptop.jpg');
  Light 1 : Subsystem
      mask Display: image('LightBulb.jpg');
  Light 2 : Subsystem
      mask Display: image('LightBulb.jpg');
  Light 3 : Subsystem
      mask Display: image('LightBulb.jpg');
  Light 4 : Subsystem
      mask Display: image('LightBulb.jpg');
  Light 5 : Subsystem
      mask Display: image('LightBulb.jpg');
  Light 6 : Subsystem
      mask Display: image('LightBulb.jpg');
  Oven : Subsystem
      mask Display: image('oven.jpg');
  Phone_Charger : Subsystem
      mask Display: image('Phone.jpg');
  Refrigerator : Subsystem
      mask Display: image('firdge1.JPG');
  Shower : Subsystem
      mask Display: image('Shower.jpg');
  Stereo : Subsystem
      mask Display: image('Stereo.jpg');
  Subsystem : Subsystem
      mask Display: patch([1 1 0 0],[1 0 0 1], [1, .4, .4])
  Subsystem1 : Subsystem
      mask Display: patch([1 1 0 0],[1 0 0 1], [0.6, .8, 1])
  Subsystem2 : Subsystem
      mask Display: patch([1 1 0 0],[1 0 0 1], [0.4, 1, .4])
  Subsystem3 : Subsystem
      mask Display: patch([1 1 0 0],[1 0 0 1], [0.8, 0.42, 0])
  Subsystem4 : Subsystem
      mask Display: patch([1 1 0 0],[1 0 0 1], [0.75, .75, .75])
  Thermostat : Subsystem
  Toaster : Subsystem
      mask Display: image('toaster.jpg');
  Tv : Subsystem
      mask Display: image('Tel.jpg');
  Water tank : Subsystem
      mask Display: image('Hot Water.jpg');
  Connection Port : PMIOPort  Side=Left
  House 4 House Power : Outport
  House 4 WH Power : Outport  Port=2
  House 4 WH Temp : Outport  Port=3
  House 4 T_High_WH : Outport  Port=4
  House 4 T_Low_WH : Outport  Port=5
  wires:
  Current Measurement1/1 -> Gain1/1
  Gain1/1 -> House 4 House Power/1
  Gain/1 -> House 4 WH Power/1
  Constant1/1 -> House 4 T_Low_WH/1
  Constant/1 -> House 4 T_High_WH/1
  Current Measurement/1 -> Gain/1
  Water tank/1(Temperature) -> Thermostat/1(In1), House 4 WH Temp/1
  Shower/1(Out1) -> Water tank/1(Mass flow rate)
  unused_solar/1 -> House 4 Controller1/2(solar)
  Thermostat/1(Out1) -> House 4 Controller1/1(thermo)
  House 4 Controller1/1(sw) -> Ideal Switch/1
  connections:
  Current Measurement1/LConn1 -- Ideal Switch/LConn1 -- Connection Port/RConn1
  Water tank/LConn1 -- Current Measurement/RConn1
  Refrigerator/LConn1 -- Kettle/LConn1 -- Toaster/LConn1 -- Light 2/LConn1 -- Light 1/LConn1 -- Oven/LConn1 -- Current Measurement1/RConn1 -- Light 3/LConn1 -- Light 4/LConn1 -- Clock 1/LConn1 -- Lamp 1/LConn1 -- Clock 2/LConn1 -- Light 5/LConn1 -- Lamp 2/LConn1 -- Laptop_Charger/RConn1 -- Laptop_Charger/LConn1 -- Phone_Charger/RConn1 -- Phone_Charger/LConn2 -- Phone_Charger/LConn1 -- Light 6/LConn1 -- Lamp 3/LConn1 -- Heater/LConn1 -- Stereo/LConn1 -- Tv/LConn1
  Ideal Switch/RConn1 -- Current Measurement/LConn1

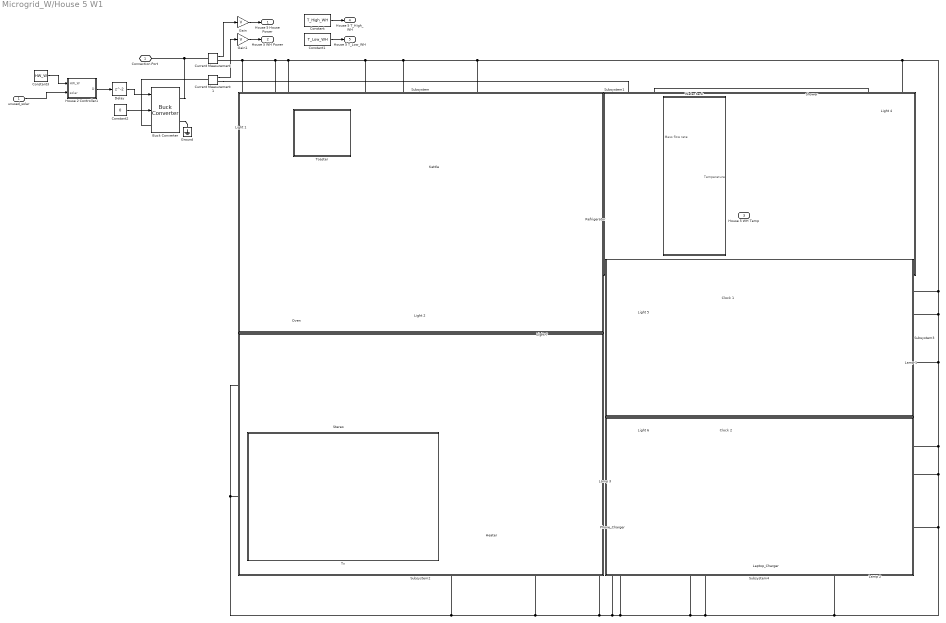
== system Microgrid_W/House 5 W1 ==
  unused_solar : Inport
  Buck Converter : powerlib/Power Electronics/Buck Converter  ModelType=Average model (D-controlled)  Ron=1e-3  Rs=1e6  Cs=inf  Vforward=[0,0]  Ron_Diode=1e-3  Rs_Diode=1e6  Cs_Diode=inf  Vf_Diode=1e-3  Rs_CurrentSource=inf
      settings: SourceProductBaseCode=PS
  Clock 1 : Subsystem
      mask Display: image('Clock.jpg');
  Clock 2 : Subsystem
      mask Display: image('Clock.jpg');
  Constant : Constant  Value=T_High_WH
  Constant1 : Constant  Value=T_Low_WH
  Constant2 : Constant  Value=0
  Constant3 : Constant  Value=HW_W
  Current Measurement : powerlib/Measurements/Current Measurement  PhasorSimulation=off  OutputType=Complex  PSBequivalent=0
  Current Measurement1 : powerlib/Measurements/Current Measurement  PhasorSimulation=off  OutputType=Complex  PSBequivalent=0
  Delay : Delay
  Gain : Gain  Gain=V
  Gain1 : Gain  Gain=V
  Ground : powerlib/Elements/Ground  LConnTagsString=a
  Heater : Subsystem
      mask Display: image('oil_heater.jpg');
  House 2 Controller1 : MATLAB Function  TreatAsAtomicUnit=on
  Kettle : Subsystem
      mask Display: image('jug.jpg');
  Lamp 1 : Subsystem
      mask Display: image('Lamp_1.jpg');
  Lamp 2 : Subsystem
      mask Display: image('Lamp_1.jpg');
  Lamp 3 : Subsystem
      mask Display: image('Lamp_1.jpg');
  Laptop_Charger : Subsystem
      mask Display: image('Laptop.jpg');
  Light 1 : Subsystem
      mask Display: image('LightBulb.jpg');
  Light 2 : Subsystem
      mask Display: image('Dishwasher.jpg');
  Light 4 : Subsystem
      mask Display: image('LightBulb.jpg');
  Light 5 : Subsystem
      mask Display: image('LightBulb.jpg');
  Light 6 : Subsystem
      mask Display: image('LightBulb.jpg');
  Light 7 : Subsystem
      mask Display: image('LightBulb.jpg');
  Oven : Subsystem
      mask Display: image('oven.jpg');
  Phone_Charger : Subsystem
      mask Display: image('Phone.jpg');
  Refrigerator : Subsystem
      mask Display: image('firdge1.JPG');
  Shower : Subsystem
      mask Display: image('Shower.jpg');
  Stereo : Subsystem
      mask Display: image('Stereo.jpg');
  Subsystem : Subsystem
      mask Display: patch([1 1 0 0],[1 0 0 1], [1, .4, .4])
  Subsystem1 : Subsystem
      mask Display: patch([1 1 0 0],[1 0 0 1], [0.6, .8, 1])
  Subsystem2 : Subsystem
      mask Display: patch([1 1 0 0],[1 0 0 1], [0.4, 1, .4])
  Subsystem3 : Subsystem
      mask Display: patch([1 1 0 0],[1 0 0 1], [0.8, 0.42, 0])
  Subsystem4 : Subsystem
      mask Display: patch([1 1 0 0],[1 0 0 1], [0.75, .75, .75])
  Toaster : Subsystem
      mask Display: image('toaster.jpg');
  Tv : Subsystem
      mask Display: image('Tel.jpg');
  Water tank : Subsystem
      mask Display: image('Hot Water.jpg');
  Connection Port : PMIOPort  Side=Left
  House 5 House Power : Outport
  House 5 WH Power : Outport  Port=2
  House 5 WH Temp : Outport  Port=3
  House 5 T_High_WH : Outport  Port=4
  House 5 T_Low_WH : Outport  Port=5
  wires:
  Shower/1(Out1) -> Water tank/1(Mass flow rate)
  Gain1/1 -> House 5 WH Power/1
  Constant/1 -> House 5 T_High_WH/1
  Constant1/1 -> House 5 T_Low_WH/1
  Water tank/1(Temperature) -> House 5 WH Temp/1
  Gain/1 -> House 5 House Power/1
  Current Measurement/1 -> Gain/1
  Current Measurement1/1 -> Gain1/1
  Constant2/1 -> Buck Converter/2
  Constant3/1 -> House 2 Controller1/1(HW_W)
  House 2 Controller1/1(D) -> Delay/1
  Delay/1 -> Buck Converter/1
  unused_solar/1 -> House 2 Controller1/2(solar)
  connections:
  Current Measurement/LConn1 -- Buck Converter/RConn1 -- Connection Port/RConn1
  Current Measurement1/RConn1 -- Water tank/LConn1
  Lamp 3/LConn1 -- Current Measurement/RConn1 -- Oven/LConn1 -- Light 1/LConn1 -- Toaster/LConn1 -- Light 2/LConn1 -- Kettle/LConn1 -- Refrigerator/LConn1 -- Light 4/LConn1 -- Light 5/LConn1 -- Clock 1/LConn1 -- Lamp 1/LConn1 -- Clock 2/LConn1 -- Light 6/LConn1 -- Lamp 2/LConn1 -- Laptop_Charger/RConn1 -- Laptop_Charger/LConn1 -- Phone_Charger/RConn1 -- Phone_Charger/LConn2 -- Phone_Charger/LConn1 -- Light 7/LConn1 -- Stereo/LConn1 -- Tv/LConn1 -- Heater/LConn1
  Buck Converter/RConn2 -- Ground/LConn1
  Buck Converter/LConn1 -- Current Measurement1/LConn1

== system Microgrid_W/House 5 W2 ==
  Clock 1 : Subsystem
      mask Display: image('Clock.jpg');
  Clock 2 : Subsystem
      mask Display: image('Clock.jpg');
  Constant : Constant  Value=T_High_WH
  Constant1 : Constant  Value=T_Low_WH
  Current Measurement : powerlib/Measurements/Current Measurement  PhasorSimulation=off  OutputType=Complex  PSBequivalent=0
  Current Measurement1 : powerlib/Measurements/Current Measurement  PhasorSimulation=off  OutputType=Complex  PSBequivalent=0
  Gain : Gain  Gain=V
  Gain1 : Gain  Gain=V
  Heater : Subsystem
      mask Display: image('oil_heater.jpg');
  Kettle : Subsystem
      mask Display: image('jug.jpg');
  Lamp 1 : Subsystem
      mask Display: image('Lamp_1.jpg');
  Lamp 2 : Subsystem
      mask Display: image('Lamp_1.jpg');
  Lamp 3 : Subsystem
      mask Display: image('Lamp_1.jpg');
  Laptop_Charger : Subsystem
      mask Display: image('Laptop.jpg');
  Light 1 : Subsystem
      mask Display: image('LightBulb.jpg');
  Light 2 : Subsystem
      mask Display: image('Dishwasher.jpg');
  Light 4 : Subsystem
      mask Display: image('LightBulb.jpg');
  Light 5 : Subsystem
      mask Display: image('LightBulb.jpg');
  Light 6 : Subsystem
      mask Display: image('LightBulb.jpg');
  Light 7 : Subsystem
      mask Display: image('LightBulb.jpg');
  Oven : Subsystem
      mask Display: image('oven.jpg');
  Phone_Charger : Subsystem
      mask Display: image('Phone.jpg');
  Refrigerator : Subsystem
      mask Display: image('firdge1.JPG');
  Shower : Subsystem
      mask Display: image('Shower.jpg');
  Stereo : Subsystem
      mask Display: image('Stereo.jpg');
  Subsystem : Subsystem
      mask Display: patch([1 1 0 0],[1 0 0 1], [1, .4, .4])
  Subsystem1 : Subsystem
      mask Display: patch([1 1 0 0],[1 0 0 1], [0.6, .8, 1])
  Subsystem2 : Subsystem
      mask Display: patch([1 1 0 0],[1 0 0 1], [0.4, 1, .4])
  Subsystem3 : Subsystem
      mask Display: patch([1 1 0 0],[1 0 0 1], [0.8, 0.42, 0])
  Subsystem4 : Subsystem
      mask Display: patch([1 1 0 0],[1 0 0 1], [0.75, .75, .75])
  Toaster : Subsystem
      mask Display: image('toaster.jpg');
  Tv : Subsystem
      mask Display: image('Tel.jpg');
  Water tank : Subsystem
      mask Display: image('Hot Water.jpg');
  Connection Port : PMIOPort  Side=Left
  House 5 House Power : Outport
  House 5 WH Power : Outport  Port=2
  House 5 WH Temp : Outport  Port=3
  House 5 T_High_WH : Outport  Port=4
  House 5 T_Low_WH : Outport  Port=5
  wires:
  Shower/1(Out1) -> Water tank/1(Mass flow rate)
  Gain1/1 -> House 5 WH Power/1
  Constant/1 -> House 5 T_High_WH/1
  Constant1/1 -> House 5 T_Low_WH/1
  Water tank/1(Temperature) -> House 5 WH Temp/1
  Gain/1 -> House 5 House Power/1
  Current Measurement/1 -> Gain/1
  Current Measurement1/1 -> Gain1/1
  connections:
  Connection Port/RConn1 -- Current Measurement/LConn1 -- Current Measurement1/LConn1
  Current Measurement1/RConn1 -- Water tank/LConn1
  Lamp 3/LConn1 -- Current Measurement/RConn1 -- Oven/LConn1 -- Light 1/LConn1 -- Toaster/LConn1 -- Light 2/LConn1 -- Kettle/LConn1 -- Refrigerator/LConn1 -- Light 4/LConn1 -- Light 5/LConn1 -- Clock 1/LConn1 -- Lamp 1/LConn1 -- Clock 2/LConn1 -- Light 6/LConn1 -- Lamp 2/LConn1 -- Laptop_Charger/RConn1 -- Laptop_Charger/LConn1 -- Phone_Charger/RConn1 -- Phone_Charger/LConn2 -- Phone_Charger/LConn1 -- Light 7/LConn1 -- Stereo/LConn1 -- Tv/LConn1 -- Heater/LConn1

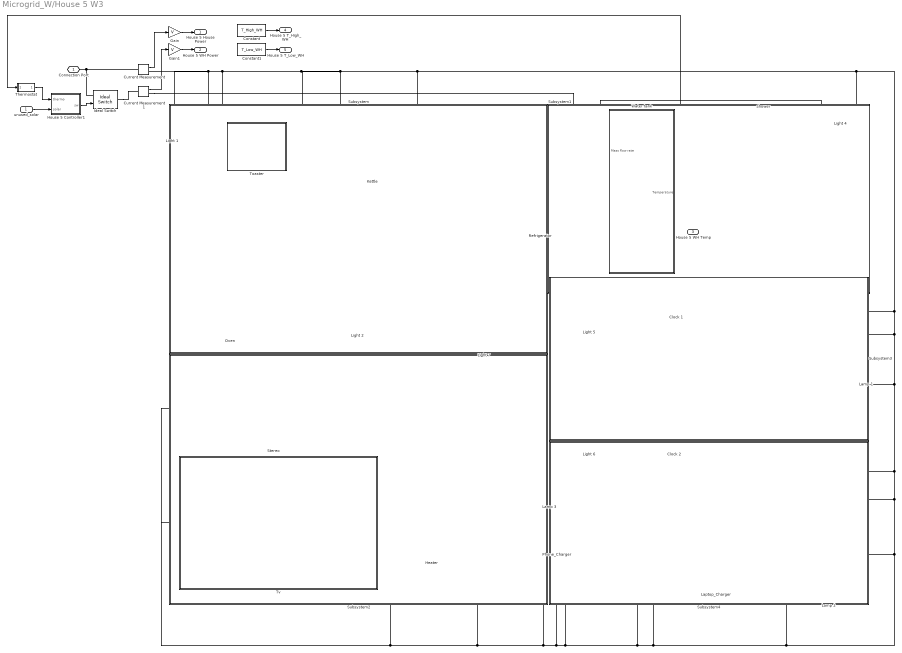
== system Microgrid_W/House 5 W3 ==
  unused_solar : Inport
  Clock 1 : Subsystem
      mask Display: image('Clock.jpg');
  Clock 2 : Subsystem
      mask Display: image('Clock.jpg');
  Constant : Constant  Value=T_High_WH
  Constant1 : Constant  Value=T_Low_WH
  Current Measurement : powerlib/Measurements/Current Measurement  PhasorSimulation=off  OutputType=Complex  PSBequivalent=0
  Current Measurement1 : powerlib/Measurements/Current Measurement  PhasorSimulation=off  OutputType=Complex  PSBequivalent=0
  Gain : Gain  Gain=V
  Gain1 : Gain  Gain=V
  Heater : Subsystem
      mask Display: image('oil_heater.jpg');
  House 5 Controller1 : MATLAB Function  TreatAsAtomicUnit=on
  Ideal Switch : powerlib/Power Electronics/Ideal Switch  Ron=0  Lon=0  IC=0  Rs=1e5  Cs=inf  Measurements=off
  Kettle : Subsystem
      mask Display: image('jug.jpg');
  Lamp 1 : Subsystem
      mask Display: image('Lamp_1.jpg');
  Lamp 2 : Subsystem
      mask Display: image('Lamp_1.jpg');
  Lamp 3 : Subsystem
      mask Display: image('Lamp_1.jpg');
  Laptop_Charger : Subsystem
      mask Display: image('Laptop.jpg');
  Light 1 : Subsystem
      mask Display: image('LightBulb.jpg');
  Light 2 : Subsystem
      mask Display: image('Dishwasher.jpg');
  Light 4 : Subsystem
      mask Display: image('LightBulb.jpg');
  Light 5 : Subsystem
      mask Display: image('LightBulb.jpg');
  Light 6 : Subsystem
      mask Display: image('LightBulb.jpg');
  Light 7 : Subsystem
      mask Display: image('LightBulb.jpg');
  Oven : Subsystem
      mask Display: image('oven.jpg');
  Phone_Charger : Subsystem
      mask Display: image('Phone.jpg');
  Refrigerator : Subsystem
      mask Display: image('firdge1.JPG');
  Shower : Subsystem
      mask Display: image('Shower.jpg');
  Stereo : Subsystem
      mask Display: image('Stereo.jpg');
  Subsystem : Subsystem
      mask Display: patch([1 1 0 0],[1 0 0 1], [1, .4, .4])
  Subsystem1 : Subsystem
      mask Display: patch([1 1 0 0],[1 0 0 1], [0.6, .8, 1])
  Subsystem2 : Subsystem
      mask Display: patch([1 1 0 0],[1 0 0 1], [0.4, 1, .4])
  Subsystem3 : Subsystem
      mask Display: patch([1 1 0 0],[1 0 0 1], [0.8, 0.42, 0])
  Subsystem4 : Subsystem
      mask Display: patch([1 1 0 0],[1 0 0 1], [0.75, .75, .75])
  Thermostat : Subsystem
  Toaster : Subsystem
      mask Display: image('toaster.jpg');
  Tv : Subsystem
      mask Display: image('Tel.jpg');
  Water tank : Subsystem
      mask Display: image('Hot Water.jpg');
  Connection Port : PMIOPort  Side=Left
  House 5 House Power : Outport
  House 5 WH Power : Outport  Port=2
  House 5 WH Temp : Outport  Port=3
  House 5 T_High_WH : Outport  Port=4
  House 5 T_Low_WH : Outport  Port=5
  wires:
  Current Measurement1/1 -> Gain1/1
  Current Measurement/1 -> Gain/1
  Gain/1 -> House 5 House Power/1
  Water tank/1(Temperature) -> Thermostat/1(In1), House 5 WH Temp/1
  Constant1/1 -> House 5 T_Low_WH/1
  Constant/1 -> House 5 T_High_WH/1
  Gain1/1 -> House 5 WH Power/1
  Shower/1(Out1) -> Water tank/1(Mass flow rate)
  unused_solar/1 -> House 5 Controller1/2(solar)
  Thermostat/1(Out1) -> House 5 Controller1/1(thermo)
  House 5 Controller1/1(sw) -> Ideal Switch/1
  connections:
  Heater/LConn1 -- Tv/LConn1 -- Stereo/LConn1 -- Light 7/LConn1 -- Phone_Charger/LConn1 -- Phone_Charger/LConn2 -- Phone_Charger/RConn1 -- Laptop_Charger/LConn1 -- Laptop_Charger/RConn1 -- Lamp 2/LConn1 -- Light 6/LConn1 -- Clock 2/LConn1 -- Lamp 1/LConn1 -- Clock 1/LConn1 -- Light 5/LConn1 -- Light 4/LConn1 -- Refrigerator/LConn1 -- Kettle/LConn1 -- Light 2/LConn1 -- Toaster/LConn1 -- Light 1/LConn1 -- Oven/LConn1 -- Current Measurement/RConn1 -- Lamp 3/LConn1
  Current Measurement1/RConn1 -- Water tank/LConn1
  Current Measurement/LConn1 -- Ideal Switch/LConn1 -- Connection Port/RConn1
  Ideal Switch/RConn1 -- Current Measurement1/LConn1

== system Microgrid_W/WH_Helper_H1 ==
  House P : Inport
  WH P : Inport  Port=2
  "BMS Bat Supply " : Inport  Port=3
  Saturation : Saturate  UpperLimit=inf  LowerLimit=0
  Saturation1 : Saturate  UpperLimit=inf  LowerLimit=0
  Subtract : Sum  Inputs=+-
  Subtract1 : Sum  Inputs=+-
  Subtract2 : Sum  Inputs=+-
  WH Bat : Outport  VectorParamsAs1DForOutWhenUnconnected=off
  House Bat : Outport  Port=2  VectorParamsAs1DForOutWhenUnconnected=off
  WH Solar : Outport  Port=3  VectorParamsAs1DForOutWhenUnconnected=off
  wires:
  Subtract2/1 -> WH Solar/1  "WH Solar"
  "BMS Bat Supply "/1 -> Subtract1/1, Subtract/1
  Subtract1/1 -> Saturation1/1
  WH P/1 -> Subtract/2, Subtract2/1
  Subtract/1 -> Saturation/1
  Saturation/1 -> House Bat/1  "House Bat"
  Saturation1/1 -> Subtract2/2, WH Bat/1  "WH Bat"
  House P/1 -> Subtract1/2

== system Microgrid_W/WH_Helper_H2 ==
  House P : Inport
  WH P : Inport  Port=2
  "BMS Bat Supply " : Inport  Port=3
  Saturation : Saturate  UpperLimit=inf  LowerLimit=0
  Saturation1 : Saturate  UpperLimit=inf  LowerLimit=0
  Subtract : Sum  Inputs=+-
  Subtract1 : Sum  Inputs=+-
  Subtract2 : Sum  Inputs=+-
  WH Bat : Outport  VectorParamsAs1DForOutWhenUnconnected=off
  House Bat : Outport  Port=2  VectorParamsAs1DForOutWhenUnconnected=off
  WH Solar : Outport  Port=3  VectorParamsAs1DForOutWhenUnconnected=off
  wires:
  House P/1 -> Subtract1/2
  Saturation1/1 -> WH Bat/1, Subtract2/2  "WH Bat"
  Saturation/1 -> House Bat/1  "House Bat"
  Subtract/1 -> Saturation/1
  WH P/1 -> Subtract2/1, Subtract/2
  Subtract1/1 -> Saturation1/1
  "BMS Bat Supply "/1 -> Subtract/1, Subtract1/1
  Subtract2/1 -> WH Solar/1  "WH Solar"

== system Microgrid_W/WH_Helper_H3 ==
  House P : Inport
  WH P : Inport  Port=2
  "BMS Bat Supply " : Inport  Port=3
  Saturation : Saturate  UpperLimit=inf  LowerLimit=0
  Saturation1 : Saturate  UpperLimit=inf  LowerLimit=0
  Subtract : Sum  Inputs=+-
  Subtract1 : Sum  Inputs=+-
  Subtract2 : Sum  Inputs=+-
  WH Bat : Outport  VectorParamsAs1DForOutWhenUnconnected=off
  House Bat : Outport  Port=2  VectorParamsAs1DForOutWhenUnconnected=off
  WH Solar : Outport  Port=3  VectorParamsAs1DForOutWhenUnconnected=off
  wires:
  Subtract2/1 -> WH Solar/1  "WH Solar"
  "BMS Bat Supply "/1 -> Subtract1/1, Subtract/1
  Subtract1/1 -> Saturation1/1
  WH P/1 -> Subtract/2, Subtract2/1
  Subtract/1 -> Saturation/1
  Saturation/1 -> House Bat/1  "House Bat"
  Saturation1/1 -> Subtract2/2, WH Bat/1  "WH Bat"
  House P/1 -> Subtract1/2

== system Microgrid_W/House 2 W1/Clock 1 ==
  Ground : powerlib/Elements/Ground  LConnTagsString=a
  Series RLC Branch2 : powerlib/Elements/Series RLC Branch  LConnTagsString=__new0  RConnTagsString=__new0  BranchType=R  Resistance=V^2/(Clock_1_W+0.000001)  Inductance=1e-3  SetiL0=off  InitialCurrent=0  Capacitance=1e-6  Setx0=off  InitialVoltage=0  Measurements=None
  + : PMIOPort  Side=Left
  connections:
  Ground/LConn1 -- Series RLC Branch2/RConn1
  +/RConn1 -- Series RLC Branch2/LConn1

== system Microgrid_W/House 2 W1/Clock 2 ==
  Ground : powerlib/Elements/Ground  LConnTagsString=a
  Series RLC Branch2 : powerlib/Elements/Series RLC Branch  LConnTagsString=__new0  RConnTagsString=__new0  BranchType=R  Resistance=V^2/(Clock_2_W+0.000001)  Inductance=1e-3  SetiL0=off  InitialCurrent=0  Capacitance=1e-6  Setx0=off  InitialVoltage=0  Measurements=None
  + : PMIOPort  Side=Left
  connections:
  Ground/LConn1 -- Series RLC Branch2/RConn1
  +/RConn1 -- Series RLC Branch2/LConn1
